simulink model "3R_Computed_Torque_Control"  (R2026a)
settings: Solver=VariableStepAuto
undefined symbols (not defined in the file): X, Y, Z
libraries: nesl_utility x37, sm_lib x29, robotcorelib x1, simulink x1
settings Model: Creator=Bosey  LastModifiedBy=Bosey

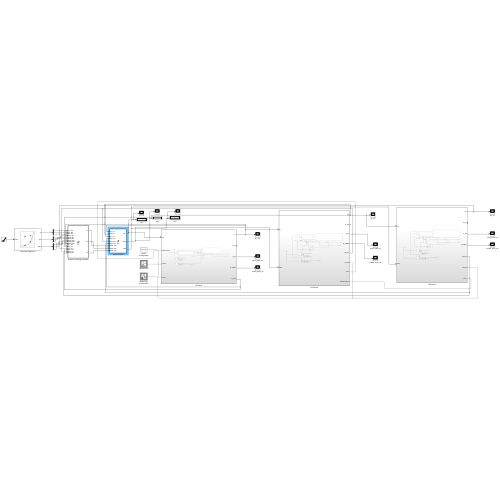
[thumbnail: Simulink's stored preview of the top-level diagram]
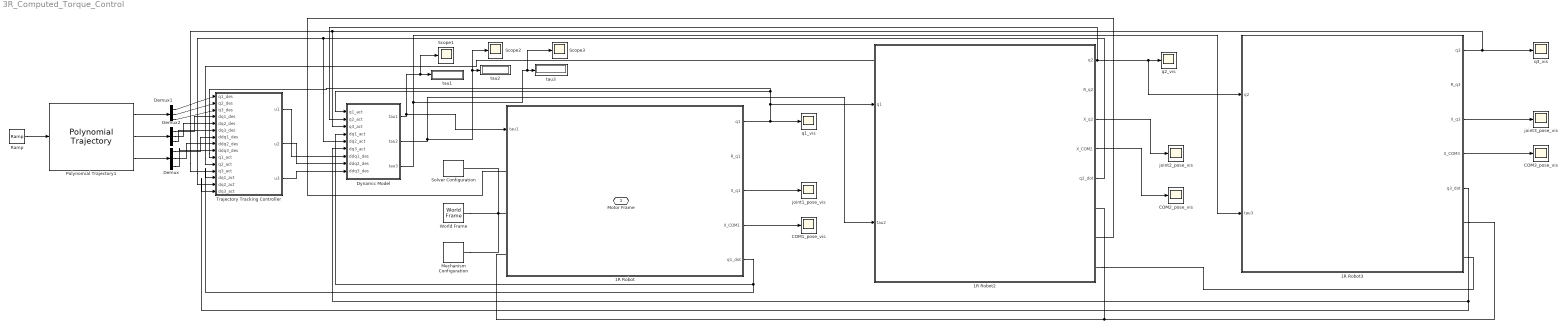
== system 3R_Computed_Torque_Control ==
  1R Robot : Subsystem
  1R Robot2 : Subsystem
  1R Robot3 : Subsystem
  COM1_pose_vis : Scope
      settings: ActiveDisplayYMinimum=-1  ActiveDisplayYMaximum=1  DataLoggingVariableName=ScopeData3
  COM2_pose_vis : Scope
      settings: DataLoggingVariableName=ScopeData5
  COM3_pose_vis : Scope
      settings: DataLoggingVariableName=ScopeData10
  Demux : Demux  Outputs=3
  Demux1 : Demux  Outputs=3
  Demux2 : Demux  Outputs=3
  Dynamic Model : MATLAB Function  TreatAsAtomicUnit=on
  Mechanism Configuration : sm_lib/Utilities/Mechanism Configuration  UniformGravity=Constant  GravityVector=[0 0 -9.80665]  GravityVectorUnits=m/s^2  LinearizationDelta=0.001  JointModeTransitionNonlinearIterations=2
  Polynomial Trajectory1 : robotcorelib/Polynomial Trajectory  WaypointSource=Internal  Waypoints=[10*pi/180, 30*pi/180; 20*pi/180, 40*pi/180; -30*pi/180, -10*pi/180]  TimePoints=[ 0, 10 ]  TimeInterval=[ 1, 4 ]  Method=Cubic Polynomial  ParameterSource=Internal  VelocityBoundaryCondition=zeros( 3, 2 )  AccelerationBoundaryCondition=zeros( 2, 5 )  SimulateUsing=Interpreted execution
  Ramp : simulink/Sources/Ramp  slope=1  start=0  InitialOutput=0
  Scope1 : Scope
      settings: ActiveDisplayYMinimum=-1  ActiveDisplayYMaximum=1  DataLoggingVariableName=ScopeData12
  Scope2 : Scope
      settings: DataLoggingVariableName=ScopeData13
  Scope3 : Scope
      settings: ActiveDisplayYMinimum=0.0024924123074908655  ActiveDisplayYMaximum=1.2543931043871539  DataLoggingVariableName=ScopeData14
  Solver Configuration : nesl_utility/Solver Configuration  PhysicalDomain=network_engine_domain  SubClassName=solver  LeftPortType=input  RightPortType=generic  Tones=[]  Harmonics=[]  SimulateNoise=off  Profile=off  UseLocalSampling=off  EnableSwitchedLinearOptims=on  FrequencyDomain=off  UseCCode=off  RelTol=0.001  AbsTol=1e-06  MinStep=1e-09  ToWorkspace=off  RevertToSquareIcSolve=off  NumHomotopyIterations=100  PhasorMode=off  PhasorModeNumHarmonics=1  ConsistencySolver=NEWTON_XTOL_AFTER_FTOL  CanonicalOrdering=UNORDERED  OptimizeIntermediates=UNOPTIMIZED  IndexReductionMethod=DerivativeReplacement  DoDC=off  ResidualTolerance=1e-09  ConsistencyTolSource=GLOBAL  ConsistencyAbsTol=0.001  ConsistencyRelTol=0.001  ConsistencyTolFactor=0.001  UseLocalSolver=off  LocalSolverChoice=NE_BACKWARD_EULER_ADVANCER  ResolveIndetEquations=on  FunctionEvalNumThread=1  LocalSolverSampleTime=0.001  DoFixedCost=off  MaxNonlinIter=3  MaxModeIter=2  ComputeImpulses=off  ImpulseIterations=2  LinearAlgebra=Sparse  LinearAlgebraNumThread=0  EquationFormulation=NE_TIME_EF  DelaysMemoryBudget=1024  AutomaticFiltering=on  FilteringTimeConstant=0.001  PartitionStorageMethod=AS_NEEDED  PartitionMemoryBudget=1024  PartitionMethod=FAST  MultibodyUseLocalSolver=off  MultibodyLocalSolverChoice=ODE1  MultibodyLocalSolverSampleTime=0.001
  Trajectory Tracking Controller : MATLAB Function  TreatAsAtomicUnit=on
  World Frame : sm_lib/Frames and Transforms/World Frame
  joint1_pose_vis : Scope
      settings: ActiveDisplayYMinimum=-1  ActiveDisplayYMaximum=1  DataLoggingVariableName=ScopeData2
  joint2_pose_vis : Scope
      settings: DataLoggingVariableName=ScopeData6
  joint3_pose_vis : Scope
      settings: DataLoggingVariableName=ScopeData9
  q1_vis : Scope
      settings: ActiveDisplayYMinimum=0.4766380114321529  ActiveDisplayYMaximum=0.5639250400174125
  q2_vis : Scope
      settings: ActiveDisplayYMinimum=0.6063223585984816  ActiveDisplayYMaximum=0.70247314524192939  DataLoggingVariableName=ScopeData4
  q3_vis : Scope
      settings: ActiveDisplayYMinimum=-0.22660836895595232  ActiveDisplayYMaximum=-0.17306799890063851  DataLoggingVariableName=ScopeData8
  tau1 : Display
  tau2 : Display
  tau3 : Display
  Motor Frame : PMIOPort  Side=Left
  wires:
  1R Robot2/1(q2) -> 1R Robot3/1(q2), q2_vis/1, Trajectory Tracking Controller/11(q2_act), Dynamic Model/2(q2_act)
  1R Robot3/4(X_COM3) -> COM3_pose_vis/1
  1R Robot2/4(X_COM2) -> COM2_pose_vis/1
  Dynamic Model/2(tau2) -> Scope2/1, tau2/1, 1R Robot2/2(tau2)
  Ramp/1 -> Polynomial Trajectory1/1
  1R Robot3/1(q3) -> Trajectory Tracking Controller/12(q3_act), Dynamic Model/3(q3_act), q3_vis/1
  1R Robot/5(q1_dot) -> Trajectory Tracking Controller/13(dq1_act), Dynamic Model/4(dq1_act)
  1R Robot3/5(q3_dot) -> Trajectory Tracking Controller/15(dq3_act), Dynamic Model/6(dq3_act)
  1R Robot3/3(X_q3) -> joint3_pose_vis/1
  1R Robot2/5(q2_dot) -> Trajectory Tracking Controller/14(dq2_act), Dynamic Model/5(dq2_act)
  1R Robot/3(X_q1) -> joint1_pose_vis/1
  1R Robot/1(q1) -> Trajectory Tracking Controller/10(q1_act), Dynamic Model/1(q1_act), 1R Robot2/1(q1), q1_vis/1
  1R Robot/4(X_COM1) -> COM1_pose_vis/1
  Dynamic Model/3(tau3) -> Scope3/1, tau3/1, 1R Robot3/2(tau3)
  1R Robot2/3(X_q2) -> joint2_pose_vis/1
  Dynamic Model/1(tau1) -> Scope1/1, tau1/1, 1R Robot/1(tau1)
  Polynomial Trajectory1/1 -> Demux1/1
  Polynomial Trajectory1/2 -> Demux2/1
  Polynomial Trajectory1/3 -> Demux/1
  Demux1/1 -> Trajectory Tracking Controller/1(q1_des)
  Demux1/2 -> Trajectory Tracking Controller/2(q2_des)
  Demux1/3 -> Trajectory Tracking Controller/3(q3_des)
  Demux2/1 -> Trajectory Tracking Controller/4(dq1_des)
  Demux2/2 -> Trajectory Tracking Controller/5(dq2_des)
  Demux2/3 -> Trajectory Tracking Controller/6(dq3_des)
  Demux/1 -> Trajectory Tracking Controller/7(ddq1_des)
  Demux/2 -> Trajectory Tracking Controller/8(ddq2_des)
  Demux/3 -> Trajectory Tracking Controller/9(ddq3_des)
  Trajectory Tracking Controller/1(u1) -> Dynamic Model/7(ddq1_des)
  Trajectory Tracking Controller/2(u2) -> Dynamic Model/8(ddq2_des)
  Trajectory Tracking Controller/3(u3) -> Dynamic Model/9(ddq3_des)
  connections:
  1R Robot2/RConn1 -- 1R Robot/LConn3 -- 1R Robot3/RConn1
  Solver Configuration/RConn1 -- Mechanism Configuration/RConn1 -- World Frame/RConn1 -- 1R Robot/LConn2
  1R Robot2/RConn3 -- 1R Robot3/RConn2
  1R Robot/LConn1 -- 1R Robot2/RConn2

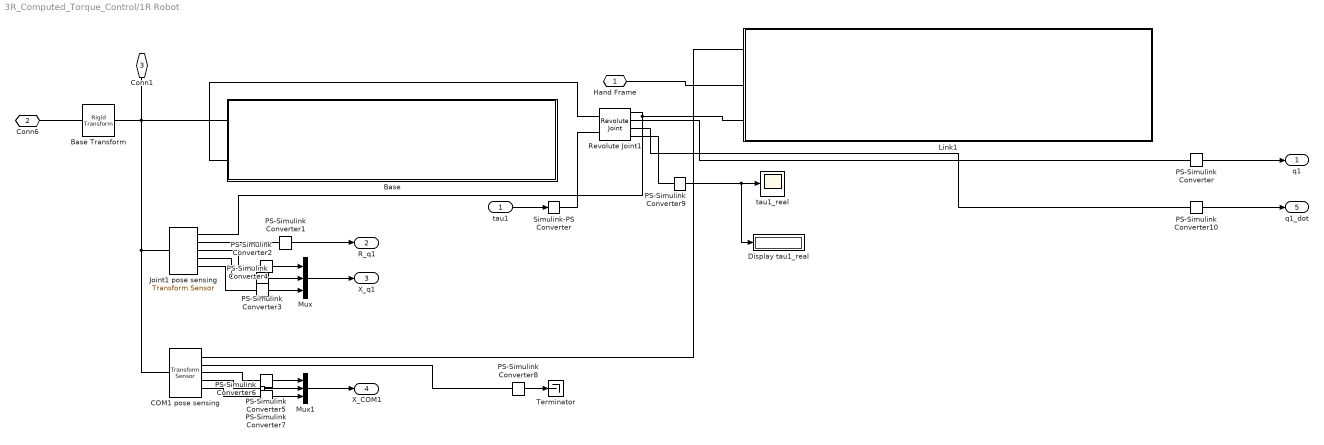
== system 3R_Computed_Torque_Control/1R Robot ==
  tau1 : Inport
  Base : Subsystem
  Base Transform : sm_lib/Frames and Transforms/Rigid Transform  RotationMethod=RotationMatrix  FollAlignAxisA=+Z  BaseAlignAxisA=-Y  FollAlignAxisB=+X  BaseAlignAxisB=+X  RotationStandardAxis=+X  RotationAngle=90  RotationAngleUnits=deg  RotationArbitraryAxis=[0 0 1]  RotationSequenceAxes=BaseAxes  RotationSequence=XYZ  RotationSequenceAngles=[90 0 0]  RotationSequenceAnglesUnits=deg  RotationMatrix=[1 0 0; 0 0 -1; 0 1 0]  Quaternion=[1 0 0 0]  TranslationMethod=None  TranslationCartesianOffset=[0 0 0]  TranslationCartesianOffsetUnits=m  TranslationStandardAxis=+Z  TranslationStandardOffset=0  TranslationStandardOffsetUnits=m  TranslationROffset=0  TranslationROffsetUnits=m  TranslationThetaOffset=0  TranslationThetaOffsetUnits=deg  TranslationZOffset=0  TranslationZOffsetUnits=m
  COM1 pose sensing : sm_lib/Frames and Transforms/Transform Sensor  MeasurementFrame=Base  RotationSequence=XYX  SenseAngle=off  SenseAxis=off  SenseQ=off  SenseR=on  SenseRotationSequence=off  SenseOmegaX=off  SenseOmegaY=off  SenseOmegaZ=off  SenseOmega=off  SenseQDot=off  SenseRDot=off  SenseRotationSequenceDot=off  SenseAlphaX=off  SenseAlphaY=off  SenseAlphaZ=off  SenseAlpha=off  SenseQDDot=off  SenseRDDot=off  SenseX=on  SenseY=on  SenseZ=on  SenseXYZ=off  SenseRad=off  SenseAzim=off  SenseDist=off  SenseInc=off  SenseXDot=off  SenseYDot=off  SenseZDot=off  SenseXYZDot=off  SenseRadDot=off  SenseAzimDot=off  SenseDistDot=off  SenseIncDot=off  SenseXDDot=off  SenseYDDot=off  SenseZDDot=off  SenseXYZDDot=off  SenseRadDDot=off  SenseAzimDDot=off  SenseDistDDot=off  SenseIncDDot=off
  Display tau1_real : Display
  Joint1 pose sensing : sm_lib/Frames and Transforms/Transform Sensor  MeasurementFrame=Base  RotationSequence=XYX  SenseAngle=off  SenseAxis=off  SenseQ=off  SenseR=on  SenseRotationSequence=off  SenseOmegaX=off  SenseOmegaY=off  SenseOmegaZ=off  SenseOmega=off  SenseQDot=off  SenseRDot=off  SenseRotationSequenceDot=off  SenseAlphaX=off  SenseAlphaY=off  SenseAlphaZ=off  SenseAlpha=off  SenseQDDot=off  SenseRDDot=off  SenseX=on  SenseY=on  SenseZ=on  SenseXYZ=off  SenseRad=off  SenseAzim=off  SenseDist=off  SenseInc=off  SenseXDot=off  SenseYDot=off  SenseZDot=off  SenseXYZDot=off  SenseRadDot=off  SenseAzimDot=off  SenseDistDot=off  SenseIncDot=off  SenseXDDot=off  SenseYDDot=off  SenseZDDot=off  SenseXYZDDot=off  SenseRadDDot=off  SenseAzimDDot=off  SenseDistDDot=off  SenseIncDDot=off
  Link1 : Subsystem
  Mux : Mux  Inputs=3
  Mux1 : Mux  Inputs=3
  PS-Simulink Converter{,1..10} (11 alike) : nesl_utility/PS-Simulink Converter  PhysicalDomain=network_engine_domain  SubClassName=ps_output  LeftPortType=input  RightPortType=output  PseudoPeriodic=off  Frequencies=[]  VectorFormat=inherit  Unit=inherit  AffineConversion=off
  Revolute Joint1 : sm_lib/Joints/Revolute Joint  JointMode=Normal  CompositeWrenchDir=FollowerOnBase  CompositeWrenchFrame=BaseFrame  SenseConstraintForce=off  SenseConstraintTorque=off  SenseTotalForce=off  SenseTotalTorque=off  PositionTargetSpecify=on  PositionTargetPriority=High  PositionTargetValue=10  PositionTargetValueUnits=deg  VelocityTargetSpecify=off  VelocityTargetPriority=High  VelocityTargetValue=0  VelocityTargetValueUnits=deg/s  EquilibriumPosition=0  EquilibriumPositionUnits=deg  SpringStiffness=0  SpringStiffnessUnits=N*m/deg  DampingCoefficient=0  DampingCoefficientUnits=N*m/(deg/s)  LowerLimitSpecify=off  LowerLimitBound=-90  LowerLimitBoundUnits=deg  LowerLimitStiffness=1e4  LowerLimitStiffnessUnits=N*m/deg  LowerLimitDamping=10  LowerLimitDampingUnits=N*m/(deg/s)  LowerLimitTransitionRegionWidth=0.1  LowerLimitTransitionRegionWidthUnits=deg  UpperLimitSpecify=off  UpperLimitBound=90  UpperLimitBoundUnits=deg  UpperLimitStiffness=1e4  UpperLimitStiffnessUnits=N*m/deg  UpperLimitDamping=10  UpperLimitDampingUnits=N*m/(deg/s)  UpperLimitTransitionRegionWidth=0.1  UpperLimitTransitionRegionWidthUnits=deg  TorqueActuationMode=InputTorque  MotionActuationMode=ComputedMotion  SensePosition=on  SenseVelocity=on  SenseAcceleration=off  SenseTorqueForce=on  SenseLowerLimitTorqueForce=off  SenseUpperLimitTorqueForce=off
  Simulink-PS Converter : nesl_utility/Simulink-PS Converter  PhysicalDomain=network_engine_domain  SubClassName=ps_input  LeftPortType=input  RightPortType=output  PseudoPeriodic=off  Frequencies=[]  NoiseDistribution=none  NoiseParameters=[]  Unit=1  AffineConversion=off  FilteringAndDerivatives=provide  SimscapeFilterOrder=1  InputFilterTimeConstant=0.001  UdotUserProvided=0
  Terminator : Terminator
  tau1_real : Scope
      settings: ActiveDisplayYMinimum=-1  ActiveDisplayYMaximum=1
  Hand Frame : PMIOPort  Side=Left
  Conn6 : PMIOPort  Port=2  Side=Left
  Conn1 : PMIOPort  Port=3  Side=Left
  q1 : Outport
  R_q1 : Outport  Port=2
  X_q1 : Outport  Port=3
  X_COM1 : Outport  Port=4
  q1_dot : Outport  Port=5
  wires:
  PS-Simulink Converter/1 -> q1/1
  tau1/1 -> Simulink-PS Converter/1
  PS-Simulink Converter1/1 -> R_q1/1
  PS-Simulink Converter2/1 -> Mux/1
  PS-Simulink Converter3/1 -> Mux/2
  PS-Simulink Converter4/1 -> Mux/3
  Mux/1 -> X_q1/1
  PS-Simulink Converter7/1 -> Mux1/3
  PS-Simulink Converter6/1 -> Mux1/2
  PS-Simulink Converter5/1 -> Mux1/1
  Mux1/1 -> X_COM1/1
  PS-Simulink Converter8/1 -> Terminator/1
  PS-Simulink Converter9/1 -> Display tau1_real/1, tau1_real/1
  PS-Simulink Converter10/1 -> q1_dot/1
  connections:
  Conn1/RConn1 -- Base/LConn1 -- Base Transform/RConn1 -- COM1 pose sensing/LConn1 -- Joint1 pose sensing/LConn1
  Base/LConn2 -- Revolute Joint1/LConn1
  Link1/LConn3 -- Joint1 pose sensing/RConn1 -- Revolute Joint1/RConn1
  COM1 pose sensing/RConn1 -- Link1/LConn1
  Revolute Joint1/RConn2 -- PS-Simulink Converter/LConn1
  Simulink-PS Converter/RConn1 -- Revolute Joint1/LConn2
  Joint1 pose sensing/RConn2 -- PS-Simulink Converter1/LConn1
  COM1 pose sensing/RConn3 -- PS-Simulink Converter5/LConn1
  COM1 pose sensing/RConn4 -- PS-Simulink Converter6/LConn1
  COM1 pose sensing/RConn5 -- PS-Simulink Converter7/LConn1
  COM1 pose sensing/RConn2 -- PS-Simulink Converter8/LConn1
  PS-Simulink Converter2/LConn1 -- Joint1 pose sensing/RConn3
  Joint1 pose sensing/RConn5 -- PS-Simulink Converter4/LConn1
  Joint1 pose sensing/RConn4 -- PS-Simulink Converter3/LConn1
  Hand Frame/RConn1 -- Link1/LConn2
  Base Transform/LConn1 -- Conn6/RConn1
  PS-Simulink Converter9/LConn1 -- Revolute Joint1/RConn4
  PS-Simulink Converter10/LConn1 -- Revolute Joint1/RConn3

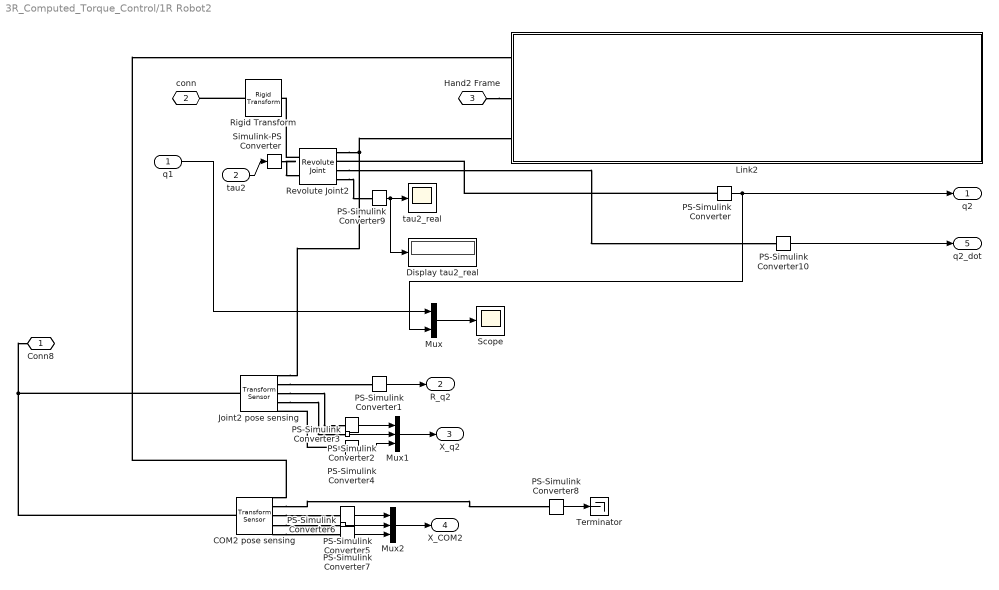
== system 3R_Computed_Torque_Control/1R Robot2 ==
  q1 : Inport
  tau2 : Inport  Port=2
  COM2 pose sensing : sm_lib/Frames and Transforms/Transform Sensor  MeasurementFrame=Base  RotationSequence=XYX  SenseAngle=off  SenseAxis=off  SenseQ=off  SenseR=on  SenseRotationSequence=off  SenseOmegaX=off  SenseOmegaY=off  SenseOmegaZ=off  SenseOmega=off  SenseQDot=off  SenseRDot=off  SenseRotationSequenceDot=off  SenseAlphaX=off  SenseAlphaY=off  SenseAlphaZ=off  SenseAlpha=off  SenseQDDot=off  SenseRDDot=off  SenseX=on  SenseY=on  SenseZ=on  SenseXYZ=off  SenseRad=off  SenseAzim=off  SenseDist=off  SenseInc=off  SenseXDot=off  SenseYDot=off  SenseZDot=off  SenseXYZDot=off  SenseRadDot=off  SenseAzimDot=off  SenseDistDot=off  SenseIncDot=off  SenseXDDot=off  SenseYDDot=off  SenseZDDot=off  SenseXYZDDot=off  SenseRadDDot=off  SenseAzimDDot=off  SenseDistDDot=off  SenseIncDDot=off
  Display tau2_real : Display
  Joint2 pose sensing : sm_lib/Frames and Transforms/Transform Sensor  MeasurementFrame=Base  RotationSequence=XYX  SenseAngle=off  SenseAxis=off  SenseQ=off  SenseR=on  SenseRotationSequence=off  SenseOmegaX=off  SenseOmegaY=off  SenseOmegaZ=off  SenseOmega=off  SenseQDot=off  SenseRDot=off  SenseRotationSequenceDot=off  SenseAlphaX=off  SenseAlphaY=off  SenseAlphaZ=off  SenseAlpha=off  SenseQDDot=off  SenseRDDot=off  SenseX=on  SenseY=on  SenseZ=on  SenseXYZ=off  SenseRad=off  SenseAzim=off  SenseDist=off  SenseInc=off  SenseXDot=off  SenseYDot=off  SenseZDot=off  SenseXYZDot=off  SenseRadDot=off  SenseAzimDot=off  SenseDistDot=off  SenseIncDot=off  SenseXDDot=off  SenseYDDot=off  SenseZDDot=off  SenseXYZDDot=off  SenseRadDDot=off  SenseAzimDDot=off  SenseDistDDot=off  SenseIncDDot=off
  Link2 : Subsystem
  Mux : Mux  Inputs=2
  Mux1 : Mux  Inputs=3
  Mux2 : Mux  Inputs=3
  PS-Simulink Converter{,1..10} (11 alike) : nesl_utility/PS-Simulink Converter  PhysicalDomain=network_engine_domain  SubClassName=ps_output  LeftPortType=input  RightPortType=output  PseudoPeriodic=off  Frequencies=[]  VectorFormat=inherit  Unit=inherit  AffineConversion=off
  Revolute Joint2 : sm_lib/Joints/Revolute Joint  JointMode=Normal  CompositeWrenchDir=FollowerOnBase  CompositeWrenchFrame=BaseFrame  SenseConstraintForce=off  SenseConstraintTorque=off  SenseTotalForce=off  SenseTotalTorque=off  PositionTargetSpecify=on  PositionTargetPriority=High  PositionTargetValue=20  PositionTargetValueUnits=deg  VelocityTargetSpecify=off  VelocityTargetPriority=High  VelocityTargetValue=0  VelocityTargetValueUnits=deg/s  EquilibriumPosition=0  EquilibriumPositionUnits=deg  SpringStiffness=0  SpringStiffnessUnits=N*m/deg  DampingCoefficient=0  DampingCoefficientUnits=N*m/(deg/s)  LowerLimitSpecify=off  LowerLimitBound=-90  LowerLimitBoundUnits=deg  LowerLimitStiffness=1e4  LowerLimitStiffnessUnits=N*m/deg  LowerLimitDamping=10  LowerLimitDampingUnits=N*m/(deg/s)  LowerLimitTransitionRegionWidth=0.1  LowerLimitTransitionRegionWidthUnits=deg  UpperLimitSpecify=off  UpperLimitBound=90  UpperLimitBoundUnits=deg  UpperLimitStiffness=1e4  UpperLimitStiffnessUnits=N*m/deg  UpperLimitDamping=10  UpperLimitDampingUnits=N*m/(deg/s)  UpperLimitTransitionRegionWidth=0.1  UpperLimitTransitionRegionWidthUnits=deg  TorqueActuationMode=InputTorque  MotionActuationMode=ComputedMotion  SensePosition=on  SenseVelocity=on  SenseAcceleration=off  SenseTorqueForce=on  SenseLowerLimitTorqueForce=off  SenseUpperLimitTorqueForce=off
  Rigid Transform : sm_lib/Frames and Transforms/Rigid Transform  RotationMethod=None  FollAlignAxisA=+X  BaseAlignAxisA=+Y  FollAlignAxisB=+Y  BaseAlignAxisB=+Z  RotationStandardAxis=+Z  RotationAngle=90  RotationAngleUnits=deg  RotationArbitraryAxis=[0 0 1]  RotationSequenceAxes=BaseAxes  RotationSequence=XYZ  RotationSequenceAngles=[-90 0 -90]  RotationSequenceAnglesUnits=deg  RotationMatrix=[1 0 0;0 1 0;0 0 1]  Quaternion=[1 0 0 0]  TranslationMethod=None  TranslationCartesianOffset=[0 0 0]  TranslationCartesianOffsetUnits=m  TranslationStandardAxis=+X  TranslationStandardOffset=0.2  TranslationStandardOffsetUnits=m  TranslationROffset=0  TranslationROffsetUnits=m  TranslationThetaOffset=0  TranslationThetaOffsetUnits=deg  TranslationZOffset=0  TranslationZOffsetUnits=m
  Scope : Scope
      settings: ActiveDisplayYMinimum=-3.9555769196396309  ActiveDisplayYMaximum=1.3121731726237904
  Simulink-PS Converter : nesl_utility/Simulink-PS Converter  PhysicalDomain=network_engine_domain  SubClassName=ps_input  LeftPortType=input  RightPortType=output  PseudoPeriodic=off  Frequencies=[]  NoiseDistribution=none  NoiseParameters=[]  Unit=1  AffineConversion=off  FilteringAndDerivatives=provide  SimscapeFilterOrder=1  InputFilterTimeConstant=0.001  UdotUserProvided=0
  Terminator : Terminator
  tau2_real : Scope
      settings: ActiveDisplayYMinimum=-1  ActiveDisplayYMaximum=1  DataLoggingVariableName=ScopeData7
  Conn8 : PMIOPort  Side=Right
  conn : PMIOPort  Port=2  Side=Right
  Hand2 Frame : PMIOPort  Port=3  Side=Right
  q2 : Outport
  R_q2 : Outport  Port=2
  X_q2 : Outport  Port=3
  X_COM2 : Outport  Port=4
  q2_dot : Outport  Port=5
  wires:
  PS-Simulink Converter8/1 -> Terminator/1
  PS-Simulink Converter4/1 -> Mux1/3
  Mux/1 -> Scope/1
  Mux1/1 -> X_q2/1
  PS-Simulink Converter2/1 -> Mux1/1
  PS-Simulink Converter7/1 -> Mux2/3
  PS-Simulink Converter3/1 -> Mux1/2
  PS-Simulink Converter1/1 -> R_q2/1
  PS-Simulink Converter6/1 -> Mux2/2
  Mux2/1 -> X_COM2/1
  PS-Simulink Converter5/1 -> Mux2/1
  q1/1 -> Mux/1
  PS-Simulink Converter9/1 -> Display tau2_real/1, tau2_real/1
  tau2/1 -> Simulink-PS Converter/1
  PS-Simulink Converter/1 -> Mux/2, q2/1
  PS-Simulink Converter10/1 -> q2_dot/1
  connections:
  PS-Simulink Converter4/LConn1 -- Joint2 pose sensing/RConn5
  COM2 pose sensing/RConn1 -- Link2/LConn1
  Revolute Joint2/RConn1 -- Joint2 pose sensing/RConn1 -- Link2/LConn3
  PS-Simulink Converter/LConn1 -- Revolute Joint2/RConn2
  Joint2 pose sensing/RConn3 -- PS-Simulink Converter2/LConn1
  Joint2 pose sensing/LConn1 -- COM2 pose sensing/LConn1 -- Conn8/RConn1
  Joint2 pose sensing/RConn2 -- PS-Simulink Converter1/LConn1
  COM2 pose sensing/RConn5 -- PS-Simulink Converter7/LConn1
  COM2 pose sensing/RConn4 -- PS-Simulink Converter6/LConn1
  COM2 pose sensing/RConn3 -- PS-Simulink Converter5/LConn1
  COM2 pose sensing/RConn2 -- PS-Simulink Converter8/LConn1
  Joint2 pose sensing/RConn4 -- PS-Simulink Converter3/LConn1
  Rigid Transform/LConn1 -- conn/RConn1
  Revolute Joint2/LConn1 -- Rigid Transform/RConn1
  Revolute Joint2/RConn4 -- PS-Simulink Converter9/LConn1
  Revolute Joint2/RConn3 -- PS-Simulink Converter10/LConn1
  Simulink-PS Converter/RConn1 -- Revolute Joint2/LConn2
  Hand2 Frame/RConn1 -- Link2/LConn2

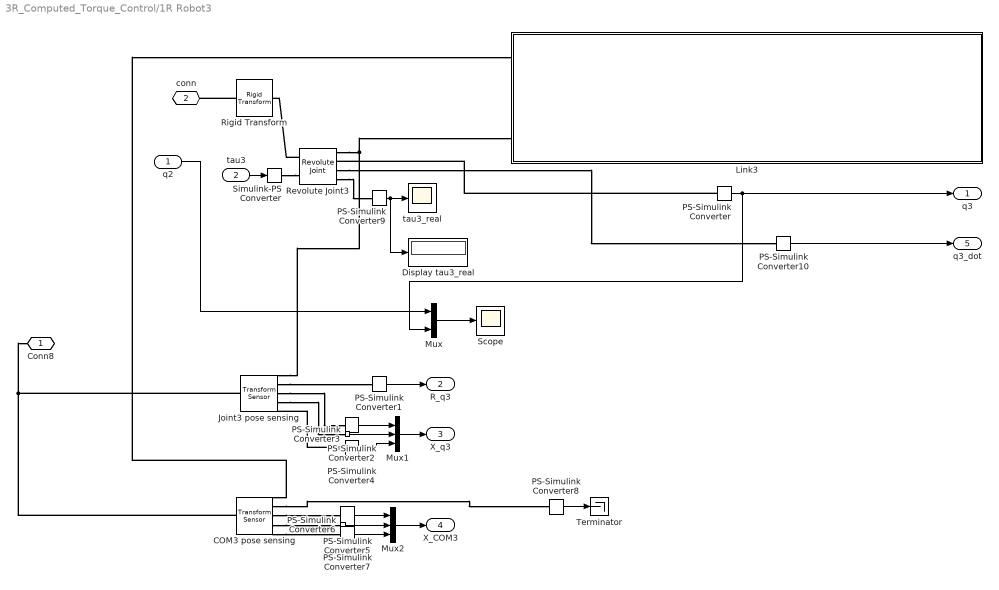
== system 3R_Computed_Torque_Control/1R Robot3 ==
  q2 : Inport
  tau3 : Inport  Port=2
  COM3 pose sensing : sm_lib/Frames and Transforms/Transform Sensor  MeasurementFrame=Base  RotationSequence=XYX  SenseAngle=off  SenseAxis=off  SenseQ=off  SenseR=on  SenseRotationSequence=off  SenseOmegaX=off  SenseOmegaY=off  SenseOmegaZ=off  SenseOmega=off  SenseQDot=off  SenseRDot=off  SenseRotationSequenceDot=off  SenseAlphaX=off  SenseAlphaY=off  SenseAlphaZ=off  SenseAlpha=off  SenseQDDot=off  SenseRDDot=off  SenseX=on  SenseY=on  SenseZ=on  SenseXYZ=off  SenseRad=off  SenseAzim=off  SenseDist=off  SenseInc=off  SenseXDot=off  SenseYDot=off  SenseZDot=off  SenseXYZDot=off  SenseRadDot=off  SenseAzimDot=off  SenseDistDot=off  SenseIncDot=off  SenseXDDot=off  SenseYDDot=off  SenseZDDot=off  SenseXYZDDot=off  SenseRadDDot=off  SenseAzimDDot=off  SenseDistDDot=off  SenseIncDDot=off
  Display tau3_real : Display
  Joint3 pose sensing : sm_lib/Frames and Transforms/Transform Sensor  MeasurementFrame=Base  RotationSequence=XYX  SenseAngle=off  SenseAxis=off  SenseQ=off  SenseR=on  SenseRotationSequence=off  SenseOmegaX=off  SenseOmegaY=off  SenseOmegaZ=off  SenseOmega=off  SenseQDot=off  SenseRDot=off  SenseRotationSequenceDot=off  SenseAlphaX=off  SenseAlphaY=off  SenseAlphaZ=off  SenseAlpha=off  SenseQDDot=off  SenseRDDot=off  SenseX=on  SenseY=on  SenseZ=on  SenseXYZ=off  SenseRad=off  SenseAzim=off  SenseDist=off  SenseInc=off  SenseXDot=off  SenseYDot=off  SenseZDot=off  SenseXYZDot=off  SenseRadDot=off  SenseAzimDot=off  SenseDistDot=off  SenseIncDot=off  SenseXDDot=off  SenseYDDot=off  SenseZDDot=off  SenseXYZDDot=off  SenseRadDDot=off  SenseAzimDDot=off  SenseDistDDot=off  SenseIncDDot=off
  Link3 : Subsystem
  Mux : Mux  Inputs=2
  Mux1 : Mux  Inputs=3
  Mux2 : Mux  Inputs=3
  PS-Simulink Converter{,1..10} (11 alike) : nesl_utility/PS-Simulink Converter  PhysicalDomain=network_engine_domain  SubClassName=ps_output  LeftPortType=input  RightPortType=output  PseudoPeriodic=off  Frequencies=[]  VectorFormat=inherit  Unit=inherit  AffineConversion=off
  Revolute Joint3 : sm_lib/Joints/Revolute Joint  JointMode=Normal  CompositeWrenchDir=FollowerOnBase  CompositeWrenchFrame=BaseFrame  SenseConstraintForce=off  SenseConstraintTorque=off  SenseTotalForce=off  SenseTotalTorque=off  PositionTargetSpecify=on  PositionTargetPriority=High  PositionTargetValue=-30  PositionTargetValueUnits=deg  VelocityTargetSpecify=off  VelocityTargetPriority=High  VelocityTargetValue=0  VelocityTargetValueUnits=deg/s  EquilibriumPosition=0  EquilibriumPositionUnits=deg  SpringStiffness=0  SpringStiffnessUnits=N*m/deg  DampingCoefficient=0  DampingCoefficientUnits=N*m/(deg/s)  LowerLimitSpecify=off  LowerLimitBound=-90  LowerLimitBoundUnits=deg  LowerLimitStiffness=1e4  LowerLimitStiffnessUnits=N*m/deg  LowerLimitDamping=10  LowerLimitDampingUnits=N*m/(deg/s)  LowerLimitTransitionRegionWidth=0.1  LowerLimitTransitionRegionWidthUnits=deg  UpperLimitSpecify=off  UpperLimitBound=90  UpperLimitBoundUnits=deg  UpperLimitStiffness=1e4  UpperLimitStiffnessUnits=N*m/deg  UpperLimitDamping=10  UpperLimitDampingUnits=N*m/(deg/s)  UpperLimitTransitionRegionWidth=0.1  UpperLimitTransitionRegionWidthUnits=deg  TorqueActuationMode=InputTorque  MotionActuationMode=ComputedMotion  SensePosition=on  SenseVelocity=on  SenseAcceleration=off  SenseTorqueForce=on  SenseLowerLimitTorqueForce=off  SenseUpperLimitTorqueForce=off
  Rigid Transform : sm_lib/Frames and Transforms/Rigid Transform  RotationMethod=None  FollAlignAxisA=+X  BaseAlignAxisA=+Y  FollAlignAxisB=+Y  BaseAlignAxisB=+Z  RotationStandardAxis=+Z  RotationAngle=90  RotationAngleUnits=deg  RotationArbitraryAxis=[0 0 1]  RotationSequenceAxes=BaseAxes  RotationSequence=XYZ  RotationSequenceAngles=[-90 0 -90]  RotationSequenceAnglesUnits=deg  RotationMatrix=[1 0 0;0 1 0;0 0 1]  Quaternion=[1 0 0 0]  TranslationMethod=None  TranslationCartesianOffset=[0 0 0]  TranslationCartesianOffsetUnits=m  TranslationStandardAxis=+X  TranslationStandardOffset=0.2  TranslationStandardOffsetUnits=m  TranslationROffset=0  TranslationROffsetUnits=m  TranslationThetaOffset=0  TranslationThetaOffsetUnits=deg  TranslationZOffset=0  TranslationZOffsetUnits=m
  Scope : Scope
      settings: ActiveDisplayYMinimum=-3.9555769196396309  ActiveDisplayYMaximum=1.3121731726237904
  Simulink-PS Converter : nesl_utility/Simulink-PS Converter  PhysicalDomain=network_engine_domain  SubClassName=ps_input  LeftPortType=input  RightPortType=output  PseudoPeriodic=off  Frequencies=[]  NoiseDistribution=none  NoiseParameters=[]  Unit=1  AffineConversion=off  FilteringAndDerivatives=provide  SimscapeFilterOrder=1  InputFilterTimeConstant=0.001  UdotUserProvided=0
  Terminator : Terminator
  tau3_real : Scope
      settings: ActiveDisplayYMinimum=0.20752725828747631  ActiveDisplayYMaximum=1.0145136066212581  DataLoggingVariableName=ScopeData7
  Conn8 : PMIOPort  Side=Right
  conn : PMIOPort  Port=2  Side=Right
  q3 : Outport
  R_q3 : Outport  Port=2
  X_q3 : Outport  Port=3
  X_COM3 : Outport  Port=4
  q3_dot : Outport  Port=5
  wires:
  PS-Simulink Converter8/1 -> Terminator/1
  PS-Simulink Converter4/1 -> Mux1/3
  Mux/1 -> Scope/1
  Mux1/1 -> X_q3/1
  PS-Simulink Converter2/1 -> Mux1/1
  PS-Simulink Converter7/1 -> Mux2/3
  PS-Simulink Converter3/1 -> Mux1/2
  PS-Simulink Converter1/1 -> R_q3/1
  PS-Simulink Converter6/1 -> Mux2/2
  Mux2/1 -> X_COM3/1
  PS-Simulink Converter5/1 -> Mux2/1
  q2/1 -> Mux/1
  PS-Simulink Converter9/1 -> Display tau3_real/1, tau3_real/1
  tau3/1 -> Simulink-PS Converter/1
  PS-Simulink Converter/1 -> Mux/2, q3/1
  PS-Simulink Converter10/1 -> q3_dot/1
  connections:
  PS-Simulink Converter4/LConn1 -- Joint3 pose sensing/RConn5
  COM3 pose sensing/RConn1 -- Link3/LConn1
  Revolute Joint3/RConn1 -- Link3/LConn3 -- Joint3 pose sensing/RConn1
  PS-Simulink Converter/LConn1 -- Revolute Joint3/RConn2
  Joint3 pose sensing/RConn3 -- PS-Simulink Converter2/LConn1
  Joint3 pose sensing/LConn1 -- COM3 pose sensing/LConn1 -- Conn8/RConn1
  Joint3 pose sensing/RConn2 -- PS-Simulink Converter1/LConn1
  COM3 pose sensing/RConn5 -- PS-Simulink Converter7/LConn1
  COM3 pose sensing/RConn4 -- PS-Simulink Converter6/LConn1
  COM3 pose sensing/RConn3 -- PS-Simulink Converter5/LConn1
  COM3 pose sensing/RConn2 -- PS-Simulink Converter8/LConn1
  Joint3 pose sensing/RConn4 -- PS-Simulink Converter3/LConn1
  Rigid Transform/LConn1 -- conn/RConn1
  Revolute Joint3/LConn1 -- Rigid Transform/RConn1
  Revolute Joint3/RConn4 -- PS-Simulink Converter9/LConn1
  Revolute Joint3/RConn3 -- PS-Simulink Converter10/LConn1
  Simulink-PS Converter/RConn1 -- Revolute Joint3/LConn2

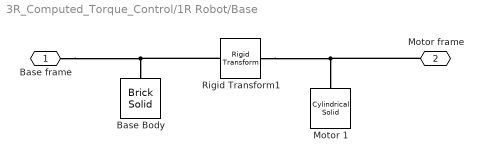
== system 3R_Computed_Torque_Control/1R Robot/Base ==
  "Base Body " : sm_lib/Body Elements/Brick Solid  BrickDimensions=[0.2 0.2 0.02]  BrickDimensionsUnits=m  ExportEntireGeometry=off  InertiaType=CalculateFromGeometry  BasedOnType=Mass  Density=1000  DensityUnits=kg/m^3  Mass=0  MassUnits=kg  CenterOfMass=[0 0 0]  CenterOfMassUnits=m  MomentsOfInertia=[1 1 1]  MomentsOfInertiaUnits=kg*m^2  ProductsOfInertia=[0 0 0]  ProductsOfInertiaUnits=kg*m^2  GraphicType=FromGeometry  MarkerShape=Sphere  MarkerSize=10  GraphicVisPropType=SimpleVisualProperties  GraphicDiffuseColor=[0.502 0.502 0.502]  GraphicOpacity=1.0  GraphicSpecularColor=[0.5 0.5 0.5 1.0]  GraphicAmbientColor=[0.15 0.15 0.15 1.0]  GraphicEmissiveColor=[0.0 0.0 0.0 1.0]  GraphicShininess=75  DoExposeReferenceFrame=on  SerializedFrames=<Frames/>
  Motor 1 : sm_lib/Body Elements/Cylindrical Solid  CylinderRadius=0.02  CylinderRadiusUnits=m  CylinderLength=0.04  CylinderLengthUnits=m  ExportEntireGeometry=off  InertiaType=CalculateFromGeometry  BasedOnType=Mass  Density=1000  DensityUnits=kg/m^3  Mass=0  MassUnits=kg  CenterOfMass=[0 0 0]  CenterOfMassUnits=m  MomentsOfInertia=[1 1 1]  MomentsOfInertiaUnits=kg*m^2  ProductsOfInertia=[0 0 0]  ProductsOfInertiaUnits=kg*m^2  GraphicType=FromGeometry  MarkerShape=Sphere  MarkerSize=10  GraphicVisPropType=SimpleVisualProperties  GraphicDiffuseColor=[0 0 0]  GraphicOpacity=1  GraphicSpecularColor=[0.5 0.5 0.5 1.0]  GraphicAmbientColor=[0.15 0.15 0.15 1.0]  GraphicEmissiveColor=[0.0 0.0 0.0 1.0]  GraphicShininess=75  DoExposeReferenceFrame=on  SerializedFrames=<Frames/>
  Rigid Transform1 : sm_lib/Frames and Transforms/Rigid Transform  RotationMethod=None  FollAlignAxisA=+X  BaseAlignAxisA=+Y  FollAlignAxisB=+Y  BaseAlignAxisB=+Z  RotationStandardAxis=+Z  RotationAngle=0  RotationAngleUnits=deg  RotationArbitraryAxis=[0 0 1]  RotationSequenceAxes=FollowerAxes  RotationSequence=XYX  RotationSequenceAngles=[0 0 0]  RotationSequenceAnglesUnits=deg  RotationMatrix=[1 0 0;0 1 0;0 0 1]  Quaternion=[1 0 0 0]  TranslationMethod=StandardAxis  TranslationCartesianOffset=[0 0 2]  TranslationCartesianOffsetUnits=m  TranslationStandardAxis=+Z  TranslationStandardOffset=0.02  TranslationStandardOffsetUnits=m  TranslationROffset=0  TranslationROffsetUnits=m  TranslationThetaOffset=0  TranslationThetaOffsetUnits=deg  TranslationZOffset=0  TranslationZOffsetUnits=m
  Base frame : PMIOPort  Side=Left
  Motor frame : PMIOPort  Port=2  Side=Left
  connections:
  Rigid Transform1/RConn1 -- Motor frame/RConn1 -- Motor 1/RConn1
  Base frame/RConn1 -- Rigid Transform1/LConn1 -- "Base Body "/RConn1

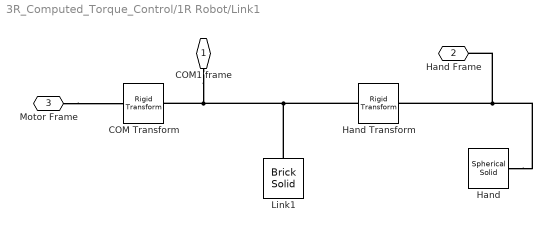
== system 3R_Computed_Torque_Control/1R Robot/Link1 ==
  COM Transform : sm_lib/Frames and Transforms/Rigid Transform  RotationMethod=None  FollAlignAxisA=+X  BaseAlignAxisA=+Y  FollAlignAxisB=+Y  BaseAlignAxisB=+Z  RotationStandardAxis=+Z  RotationAngle=0  RotationAngleUnits=deg  RotationArbitraryAxis=[0 0 1]  RotationSequenceAxes=FollowerAxes  RotationSequence=XYX  RotationSequenceAngles=[0 0 0]  RotationSequenceAnglesUnits=deg  RotationMatrix=[1 0 0;0 1 0;0 0 1]  Quaternion=[1 0 0 0]  TranslationMethod=StandardAxis  TranslationCartesianOffset=[0 0 0]  TranslationCartesianOffsetUnits=m  TranslationStandardAxis=+X  TranslationStandardOffset=0.1  TranslationStandardOffsetUnits=m  TranslationROffset=0  TranslationROffsetUnits=m  TranslationThetaOffset=0  TranslationThetaOffsetUnits=deg  TranslationZOffset=0  TranslationZOffsetUnits=m
  Hand Transform : sm_lib/Frames and Transforms/Rigid Transform  RotationMethod=None  FollAlignAxisA=+Z  BaseAlignAxisA=+X  FollAlignAxisB=+Y  BaseAlignAxisB=-Z  RotationStandardAxis=+Z  RotationAngle=0  RotationAngleUnits=deg  RotationArbitraryAxis=[0 0 1]  RotationSequenceAxes=FollowerAxes  RotationSequence=XYX  RotationSequenceAngles=[0 0 0]  RotationSequenceAnglesUnits=deg  RotationMatrix=[1 0 0;0 1 0;0 0 1]  Quaternion=[1 0 0 0]  TranslationMethod=StandardAxis  TranslationCartesianOffset=[0 0 0]  TranslationCartesianOffsetUnits=m  TranslationStandardAxis=+X  TranslationStandardOffset=0.1  TranslationStandardOffsetUnits=m  TranslationROffset=0  TranslationROffsetUnits=m  TranslationThetaOffset=0  TranslationThetaOffsetUnits=deg  TranslationZOffset=0  TranslationZOffsetUnits=m
  "Hand " : sm_lib/Body Elements/Spherical Solid  SphereRadius=0.01  SphereRadiusUnits=m  ExportEntireGeometry=off  InertiaType=CalculateFromGeometry  BasedOnType=Mass  Density=1000  DensityUnits=kg/m^3  Mass=0  MassUnits=kg  CenterOfMass=[0 0 0]  CenterOfMassUnits=m  MomentsOfInertia=[1 1 1]  MomentsOfInertiaUnits=kg*m^2  ProductsOfInertia=[0 0 0]  ProductsOfInertiaUnits=kg*m^2  GraphicType=FromGeometry  MarkerShape=Sphere  MarkerSize=10  GraphicVisPropType=SimpleVisualProperties  GraphicDiffuseColor=[0.04314 0 0.502]  GraphicOpacity=1  GraphicSpecularColor=[0.5 0.5 0.5 1.0]  GraphicAmbientColor=[0.15 0.15 0.15 1.0]  GraphicEmissiveColor=[0.0 0.0 0.0 1.0]  GraphicShininess=75  DoExposeReferenceFrame=on  SerializedFrames=<Frames/>
  Link1 : sm_lib/Body Elements/Brick Solid  BrickDimensions=[0.2 0.01 0.01]  BrickDimensionsUnits=m  ExportEntireGeometry=off  InertiaType=CalculateFromGeometry  BasedOnType=Mass  Density=1000  DensityUnits=kg/m^3  Mass=2.5  MassUnits=kg  CenterOfMass=[0 0 0]  CenterOfMassUnits=m  MomentsOfInertia=[1 1 1]  MomentsOfInertiaUnits=kg*m^2  ProductsOfInertia=[0 0 0]  ProductsOfInertiaUnits=kg*m^2  GraphicType=FromGeometry  MarkerShape=Sphere  MarkerSize=10  GraphicVisPropType=SimpleVisualProperties  GraphicDiffuseColor=[0.6667 0 0]  GraphicOpacity=1  GraphicSpecularColor=[0.5 0.5 0.5 1.0]  GraphicAmbientColor=[0.15 0.15 0.15 1.0]  GraphicEmissiveColor=[0.0 0.0 0.0 1.0]  GraphicShininess=75  DoExposeReferenceFrame=on  SerializedFrames=<Frames/>
  COM1 frame : PMIOPort  Side=Left
  Hand Frame : PMIOPort  Port=2  Side=Left
  Motor Frame : PMIOPort  Port=3  Side=Left
  connections:
  "Hand "/RConn1 -- Hand Frame/RConn1 -- Hand Transform/RConn1
  Link1/RConn1 -- Hand Transform/LConn1 -- COM Transform/RConn1 -- COM1 frame/RConn1
  Motor Frame/RConn1 -- COM Transform/LConn1

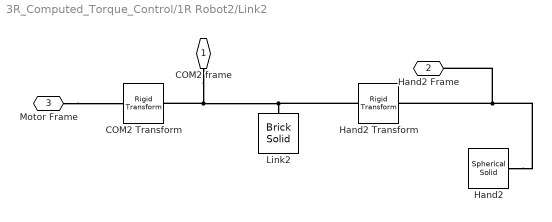
== system 3R_Computed_Torque_Control/1R Robot2/Link2 ==
  COM2 Transform : sm_lib/Frames and Transforms/Rigid Transform  RotationMethod=None  FollAlignAxisA=+X  BaseAlignAxisA=+Y  FollAlignAxisB=+Y  BaseAlignAxisB=+Z  RotationStandardAxis=+Z  RotationAngle=-90  RotationAngleUnits=deg  RotationArbitraryAxis=[0 0 1]  RotationSequenceAxes=FollowerAxes  RotationSequence=XYX  RotationSequenceAngles=[0 0 0]  RotationSequenceAnglesUnits=deg  RotationMatrix=[1 0 0;0 1 0;0 0 1]  Quaternion=[1 0 0 0]  TranslationMethod=StandardAxis  TranslationCartesianOffset=[0 0 0]  TranslationCartesianOffsetUnits=m  TranslationStandardAxis=+X  TranslationStandardOffset=0.1  TranslationStandardOffsetUnits=m  TranslationROffset=0  TranslationROffsetUnits=m  TranslationThetaOffset=0  TranslationThetaOffsetUnits=deg  TranslationZOffset=0  TranslationZOffsetUnits=m
  Hand2 Transform : sm_lib/Frames and Transforms/Rigid Transform  RotationMethod=None  FollAlignAxisA=+X  BaseAlignAxisA=+Y  FollAlignAxisB=+Y  BaseAlignAxisB=+Z  RotationStandardAxis=+Z  RotationAngle=0  RotationAngleUnits=deg  RotationArbitraryAxis=[0 0 1]  RotationSequenceAxes=FollowerAxes  RotationSequence=XYX  RotationSequenceAngles=[0 0 0]  RotationSequenceAnglesUnits=deg  RotationMatrix=[1 0 0;0 1 0;0 0 1]  Quaternion=[1 0 0 0]  TranslationMethod=StandardAxis  TranslationCartesianOffset=[0 0 0]  TranslationCartesianOffsetUnits=m  TranslationStandardAxis=+X  TranslationStandardOffset=0.1  TranslationStandardOffsetUnits=m  TranslationROffset=0  TranslationROffsetUnits=m  TranslationThetaOffset=0  TranslationThetaOffsetUnits=deg  TranslationZOffset=0  TranslationZOffsetUnits=m
  "Hand2 " : sm_lib/Body Elements/Spherical Solid  SphereRadius=0.01  SphereRadiusUnits=m  ExportEntireGeometry=off  InertiaType=CalculateFromGeometry  BasedOnType=Mass  Density=1000  DensityUnits=kg/m^3  Mass=0  MassUnits=kg  CenterOfMass=[0 0 0]  CenterOfMassUnits=m  MomentsOfInertia=[1 1 1]  MomentsOfInertiaUnits=kg*m^2  ProductsOfInertia=[0 0 0]  ProductsOfInertiaUnits=kg*m^2  GraphicType=FromGeometry  MarkerShape=Sphere  MarkerSize=10  GraphicVisPropType=SimpleVisualProperties  GraphicDiffuseColor=[0.04314 0 0.502]  GraphicOpacity=1  GraphicSpecularColor=[0.5 0.5 0.5 1.0]  GraphicAmbientColor=[0.15 0.15 0.15 1.0]  GraphicEmissiveColor=[0.0 0.0 0.0 1.0]  GraphicShininess=75  DoExposeReferenceFrame=on  SerializedFrames=<Frames/>
  Link2 : sm_lib/Body Elements/Brick Solid  BrickDimensions=[0.2 0.01 0.01]  BrickDimensionsUnits=m  ExportEntireGeometry=off  InertiaType=CalculateFromGeometry  BasedOnType=Mass  Density=1000  DensityUnits=kg/m^3  Mass=4.5  MassUnits=kg  CenterOfMass=[0 0 0]  CenterOfMassUnits=m  MomentsOfInertia=[1 1 1]  MomentsOfInertiaUnits=kg*m^2  ProductsOfInertia=[0 0 0]  ProductsOfInertiaUnits=kg*m^2  GraphicType=FromGeometry  MarkerShape=Sphere  MarkerSize=10  GraphicVisPropType=SimpleVisualProperties  GraphicDiffuseColor=[0.6667 0 0]  GraphicOpacity=1  GraphicSpecularColor=[0.5 0.5 0.5 1.0]  GraphicAmbientColor=[0.15 0.15 0.15 1.0]  GraphicEmissiveColor=[0.0 0.0 0.0 1.0]  GraphicShininess=75  DoExposeReferenceFrame=on  SerializedFrames=<Frames/>
  COM2 frame : PMIOPort  Side=Left
  Hand2 Frame : PMIOPort  Port=2  Side=Left
  Motor Frame : PMIOPort  Port=3  Side=Left
  connections:
  Hand2 Transform/RConn1 -- "Hand2 "/RConn1 -- Hand2 Frame/RConn1
  Hand2 Transform/LConn1 -- Link2/RConn1 -- COM2 Transform/RConn1 -- COM2 frame/RConn1
  Motor Frame/RConn1 -- COM2 Transform/LConn1

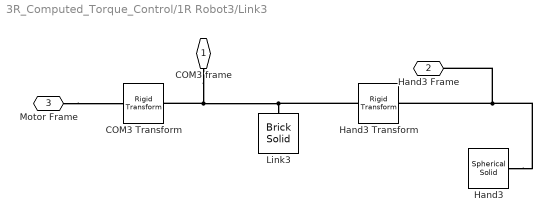
== system 3R_Computed_Torque_Control/1R Robot3/Link3 ==
  COM3 Transform : sm_lib/Frames and Transforms/Rigid Transform  RotationMethod=None  FollAlignAxisA=+X  BaseAlignAxisA=+Y  FollAlignAxisB=+Y  BaseAlignAxisB=+Z  RotationStandardAxis=+Z  RotationAngle=-90  RotationAngleUnits=deg  RotationArbitraryAxis=[0 0 1]  RotationSequenceAxes=FollowerAxes  RotationSequence=XYX  RotationSequenceAngles=[0 0 0]  RotationSequenceAnglesUnits=deg  RotationMatrix=[1 0 0;0 1 0;0 0 1]  Quaternion=[1 0 0 0]  TranslationMethod=StandardAxis  TranslationCartesianOffset=[0 0 0]  TranslationCartesianOffsetUnits=m  TranslationStandardAxis=+X  TranslationStandardOffset=0.1  TranslationStandardOffsetUnits=m  TranslationROffset=0  TranslationROffsetUnits=m  TranslationThetaOffset=0  TranslationThetaOffsetUnits=deg  TranslationZOffset=0  TranslationZOffsetUnits=m
  Hand3 Transform : sm_lib/Frames and Transforms/Rigid Transform  RotationMethod=None  FollAlignAxisA=+X  BaseAlignAxisA=+Y  FollAlignAxisB=+Y  BaseAlignAxisB=+Z  RotationStandardAxis=+Z  RotationAngle=0  RotationAngleUnits=deg  RotationArbitraryAxis=[0 0 1]  RotationSequenceAxes=FollowerAxes  RotationSequence=XYX  RotationSequenceAngles=[0 0 0]  RotationSequenceAnglesUnits=deg  RotationMatrix=[1 0 0;0 1 0;0 0 1]  Quaternion=[1 0 0 0]  TranslationMethod=StandardAxis  TranslationCartesianOffset=[0 0 0]  TranslationCartesianOffsetUnits=m  TranslationStandardAxis=+X  TranslationStandardOffset=0.1  TranslationStandardOffsetUnits=m  TranslationROffset=0  TranslationROffsetUnits=m  TranslationThetaOffset=0  TranslationThetaOffsetUnits=deg  TranslationZOffset=0  TranslationZOffsetUnits=m
  "Hand3 " : sm_lib/Body Elements/Spherical Solid  SphereRadius=0.01  SphereRadiusUnits=m  ExportEntireGeometry=off  InertiaType=CalculateFromGeometry  BasedOnType=Mass  Density=1000  DensityUnits=kg/m^3  Mass=0  MassUnits=kg  CenterOfMass=[0 0 0]  CenterOfMassUnits=m  MomentsOfInertia=[1 1 1]  MomentsOfInertiaUnits=kg*m^2  ProductsOfInertia=[0 0 0]  ProductsOfInertiaUnits=kg*m^2  GraphicType=FromGeometry  MarkerShape=Sphere  MarkerSize=10  GraphicVisPropType=SimpleVisualProperties  GraphicDiffuseColor=[0.04314 0 0.502]  GraphicOpacity=1  GraphicSpecularColor=[0.5 0.5 0.5 1.0]  GraphicAmbientColor=[0.15 0.15 0.15 1.0]  GraphicEmissiveColor=[0.0 0.0 0.0 1.0]  GraphicShininess=75  DoExposeReferenceFrame=on  SerializedFrames=<Frames/>
  Link3 : sm_lib/Body Elements/Brick Solid  BrickDimensions=[0.2 0.01 0.01]  BrickDimensionsUnits=m  ExportEntireGeometry=off  InertiaType=CalculateFromGeometry  BasedOnType=Mass  Density=1000  DensityUnits=kg/m^3  Mass=1.5  MassUnits=kg  CenterOfMass=[0 0 0]  CenterOfMassUnits=m  MomentsOfInertia=[1 1 1]  MomentsOfInertiaUnits=kg*m^2  ProductsOfInertia=[0 0 0]  ProductsOfInertiaUnits=kg*m^2  GraphicType=FromGeometry  MarkerShape=Sphere  MarkerSize=10  GraphicVisPropType=SimpleVisualProperties  GraphicDiffuseColor=[0.6667 0 0]  GraphicOpacity=1  GraphicSpecularColor=[0.5 0.5 0.5 1.0]  GraphicAmbientColor=[0.15 0.15 0.15 1.0]  GraphicEmissiveColor=[0.0 0.0 0.0 1.0]  GraphicShininess=75  DoExposeReferenceFrame=on  SerializedFrames=<Frames/>
  COM3 frame : PMIOPort  Side=Left
  Hand3 Frame : PMIOPort  Port=2  Side=Left
  Motor Frame : PMIOPort  Port=3  Side=Left
  connections:
  Hand3 Transform/RConn1 -- "Hand3 "/RConn1 -- Hand3 Frame/RConn1
  Hand3 Transform/LConn1 -- Link3/RConn1 -- COM3 Transform/RConn1 -- COM3 frame/RConn1
  Motor Frame/RConn1 -- COM3 Transform/LConn1

== matlab function 3R_Computed_Torque_Control/Dynamic Model ==
  data: q1_act input; q2_act input; q3_act input; dq1_act input; dq2_act input; dq3_act input; tau1 output; ddq1_des input; ddq2_des input; tau2 output; ddq3_des input; tau3 output
function [tau1, tau2, tau3] = fcn(q1_act, q2_act, q3_act, dq1_act, dq2_act, dq3_act, ddq1_des, ddq2_des, ddq3_des)

    %% ROBOT PARAMETERS & INITIALIZATION
    n = 3; 
    g = 9.80665;
    
    % input vectors
    q_act   = [q1_act; q2_act; q3_act];
    dq_act  = [dq1_act; dq2_act; dq3_act];
    ddq_des = [ddq1_des; ddq2_des; ddq3_des];
    l = [0.2, 0.2, 0.2]; 
    m = [2.5, 4.5, 1.5]; 
    
    % Pre-allocate data structures
    w  = zeros(3, n+1);  
    dw = zeros(3, n+1);  
    dv = zeros(3, n+1);  
    dvc = zeros(3, n);   
    F   = zeros(3, n);   
    N   = zeros(3, n);   
    f   = zeros(3, n+1); 
    nn  = zeros(3, n+1); 
    tau = zeros(n, 1);   
    
    % Local Geometry definitions
    Z = [0; 0; 1];       
    P = zeros(3, n);     
    P_com = zeros(3, n); 
    I = zeros(3, 3, n);  
    
    for i = 1:n
        P(:, i) = [l(i); 0; 0];
        P_com(:, i) = [l(i)/2; 0; 0];
        iz = (1/12) * m(i) * l(i)^2;
        I(:, :, i) = diag([0, 0, iz]);
    end

    % PURE PLANAR ROTATION MATRICES
    R_link = zeros(3, 3, n);
    
    % Link 1 Rotation 
    c1 = cos(q_act(1)); s1 = sin(q_act(1));
    R_link(:,:,1) = [c1 -s1 0; s1 c1 0; 0 0 1];
    
    % Link 2 Rotation 
    c2 = cos(q_act(2)); s2 = sin(q_act(2));
    R_link(:,:,2) = [c2 -s2 0; s2 c2 0; 0 0 1];

    % Link 3 Rotation 
    c3 = cos(q_act(3)); s3 = sin(q_act(3));
    R_link(:,:,3) = [c3 -s3 0; s3 c3 0; 0 0 1];

    % Base Boundary Conditions 
    w(:, 1)  = [0; 0; 0];
    dw(:, 1) = [0; 0; 0];
    dv(:, 1) = [0; g; 0]; 

    %% FORWARD RECURSION (i = 1 to n)
    for i = 1:n
        R_prev_to_curr = R_link(:,:,i)'; 
        
        % Angular Velocity
        w(:, i+1) = R_prev_to_curr * w(:, i) + dq_act(i) * Z;
        
        % Angular Acceleration
        dw(:, i+1) = R_prev_to_curr * dw(:, i) + ...
                     cross(R_prev_to_curr * w(:, i), dq_act(i) * Z) + ...
                     ddq_des(i) * Z;
        
        % Linear Acceleration of Joint Origin
        dv(:, i+1) = R_prev_to_curr * (dw(:, i) + cross(dw(:, i), P(:, i)) + ...
                     cross(w(:, i), cross(w(:, i), P(:, i))) + dv(:, i));
        
        % Linear Acceleration of COM
        dvc(:, i) = cross(dw(:, i+1), P_com(:, i)) + ...
                    cross(w(:, i+1), cross(w(:, i+1), P_com(:, i))) + ...
                    dv(:, i+1);
        
        % Force and Torque acting on COM
        F(:, i) = m(i) * dvc(:, i);
        N(:, i) = I(:,:,i) * dw(:, i+1) + cross(w(:, i+1), I(:,:,i) * w(:, i+1));
    end

    %% BACKWARD RECURSION (i = n down to 1)
    f(:, n+1) = [0; 0; 0];
    nn(:, n+1) = [0; 0; 0];
    
    for i = n:-1:1
        if i == n
            R_curr_to_next = eye(3);
            P_curr_to_next = [0; 0; 0];
        else
            R_curr_to_next = R_link(:,:,i+1);
            P_curr_to_next = P(:, i+1);
        end
        
        % Force acting on Joint
        f(:, i) = R_curr_to_next * f(:, i+1) + F(:, i);
        
        % Torque acting on Joint
        nn(:, i) = N(:, i) + R_curr_to_next * nn(:, i+1) + ...
                   cross(P_com(:, i), F(:, i)) + ...
                   cross(P_curr_to_next, R_curr_to_next * f(:, i+1));
        
        % Torque projection onto Joint motion axis
        tau(i) = nn(:, i)' * Z;
    end
    
    tau1 = tau(1);
    tau2 = tau(2);
    tau3 = tau(3);
   
end

== matlab function 3R_Computed_Torque_Control/Trajectory Tracking Controller ==
  data: q1_des input; u1 output; q2_des input; q3_des input; dq1_des input; dq2_des input; dq3_des input; ddq1_des input; ddq2_des input; ddq3_des input; q1_act input; q2_act input; q3_act input; dq1_act input; dq2_act input; u2 output; dq3_act input; u3 output
function [u1, u2, u3] = fcn(q1_des, q2_des, q3_des, dq1_des, dq2_des, dq3_des, ddq1_des, ddq2_des, ddq3_des, q1_act, q2_act, q3_act, dq1_act, dq2_act, dq3_act)
    % Control Gains 
    Kp = 5; 
    Kd = 4.5;

    % Calculate auxiliary acceleration 
    u1 = ddq1_des + Kp * (q1_des - q1_act) + Kd * (dq1_des - dq1_act);
    u2 = ddq2_des + Kp * (q2_des - q2_act) + Kd * (dq2_des - dq2_act);
    u3 = ddq3_des + Kp * (q3_des - q3_act) + Kd * (dq3_des - dq3_act);
end
